simulink model "pidCascadeTuner"  (Simulink 8.1)
settings: Solver=ode15s  StartTime=0.0  StopTime=20*3600  MaxStep=1  MinStep=1e-14  RelTol=1e-10  AbsTol=1e-10
settings Model: Creator=Administrator  LastModifiedBy=Administrator
settings SolverCC: InitialStep=1e-14
settings DataIOCC: SignalLoggingSaveFormat=Dataset
settings OptimizationCC: ExpressionDepthLimit=128
settings DebuggingCC: FcnCallInpInsideContextMsg=EnableAllAsError
settings GRTTargetCC: CombineOutputUpdateFcns=on  GRTInterface=off

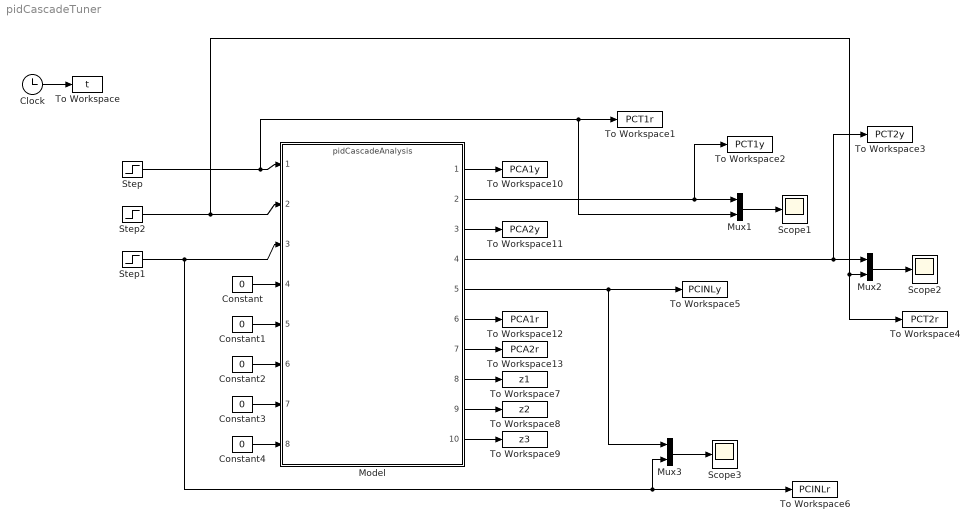
== system pidCascadeTuner ==
  Clock : Clock
  Constant{,1..4} (5 alike) : Constant  Value=0
  Model : ModelReference  ModelNameDialog=pidCascadeAnalysis  SimulationMode=Normal  ModelReferenceVersion=1.76  CopyOfModelName=pidCascadeAnalysis  DefaultDataLogging=on
  Mux1 : Mux  Inputs=2
  Mux2 : Mux  Inputs=2
  Mux3 : Mux  Inputs=2
  Scope1 : Scope
  Scope2 : Scope
  Scope3 : Scope
      settings: SaveName=ScopeData2
  Step : Step  Time=5*3600  After=-1e5  SampleTime=0
  Step1 : Step  Time=15*3600  After=-1e5  SampleTime=0
  Step2 : Step  Time=10*3600  After=-1e5  SampleTime=0
  To Workspace : ToWorkspace  VariableName=t  SampleTime=-1
  To Workspace1 : ToWorkspace  VariableName=PCT1r  SampleTime=-1
  To Workspace10 : ToWorkspace  VariableName=PCA1y  SampleTime=-1
  To Workspace11 : ToWorkspace  VariableName=PCA2y  SampleTime=-1
  To Workspace12 : ToWorkspace  VariableName=PCA1r  SampleTime=-1
  To Workspace13 : ToWorkspace  VariableName=PCA2r  SampleTime=-1
  To Workspace2 : ToWorkspace  VariableName=PCT1y  SampleTime=-1
  To Workspace3 : ToWorkspace  VariableName=PCT2y  SampleTime=-1
  To Workspace4 : ToWorkspace  VariableName=PCT2r  SampleTime=-1
  To Workspace5 : ToWorkspace  VariableName=PCINLy  SampleTime=-1
  To Workspace6 : ToWorkspace  VariableName=PCINLr  SampleTime=-1
  To Workspace7 : ToWorkspace  VariableName=z1  SampleTime=-1
  To Workspace8 : ToWorkspace  VariableName=z2  SampleTime=-1
  To Workspace9 : ToWorkspace  VariableName=z3  SampleTime=-1
  wires:
  Model/2 -> To Workspace2/1, Mux1/1
  Model/4 -> To Workspace3/1, Mux2/1
  Step/1 -> To Workspace1/1, Mux1/2, Model/1
  Step2/1 -> To Workspace4/1, Mux2/2, Model/2
  Step1/1 -> To Workspace6/1, Mux3/2, Model/3
  Mux1/1 -> Scope1/1
  Mux2/1 -> Scope2/1
  Clock/1 -> To Workspace/1
  Mux3/1 -> Scope3/1
  Model/10 -> To Workspace9/1
  Model/9 -> To Workspace8/1
  Model/8 -> To Workspace7/1
  Model/5 -> To Workspace5/1, Mux3/1
  Constant/1 -> Model/4
  Constant1/1 -> Model/5
  Constant2/1 -> Model/6
  Constant3/1 -> Model/7
  Model/1 -> To Workspace10/1
  Model/3 -> To Workspace11/1
  Model/6 -> To Workspace12/1
  Model/7 -> To Workspace13/1
  Constant4/1 -> Model/8
